simulink model "CH4_3"  (Simulink 5.0)
settings: Solver=ode23tb  SolverMode=SingleTasking  StartTime=0.0  StopTime=8/60  FixedStep=100e-6  RelTol=1e-3  AbsTol=1e-2
libraries: powerlib2 x15, powerlib_extras x6
Description:
  | 高苑科技大學 電機系
  | 電力電子實驗室
settings Model: Creator=徐瑞隆老師  LastModifiedBy=ELECTRONIC  ExtModeTrigMode=oneshot  ExtModeArmWhenConnect=off  SaveTime=off  TimeSaveName=t  SaveOutput=off  LimitDataPoints=off  BlockReductionOpt=off  BooleanDataType=off  RTWTemplateMakefile=grt_unix.tmf

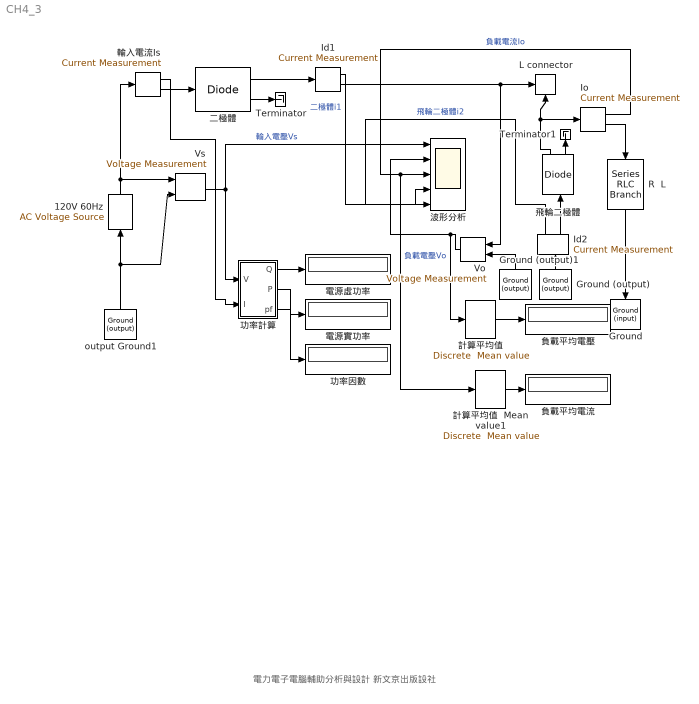
== system CH4_3 ==
  note: 電力電子電腦輔助分析與設計 新文京出版設社
  120V 60Hz : powerlib2/Electrical Sources/AC Voltage Source  Tag=PoWeRsYsTeMbLoCk  Orientation=up  A=120*1.414  P=0  F=60  stime=0  mesure=None  PSBOutputType=1
  Ground : powerlib2/Connectors/Ground (input)  Tag=PoWeRsYsTeMbLoCk  Orientation=down
  Ground (output) : powerlib2/Connectors/Ground (output)  Tag=PoWeRsYsTeMbLoCk  Orientation=up  PSBOutputType=1
  Ground (output)1 : powerlib2/Connectors/Ground (output)  Tag=PoWeRsYsTeMbLoCk  Orientation=up  PSBOutputType=1
  Id1 : powerlib2/Measurements/Current Measurement  Tag=PoWeRsYsTeMmEaSuReMeNt  PhasorSimulation=off  OutputType=Magnitude  PSBOutputType=01  PSBequivalent=0
  Id2 : powerlib2/Measurements/Current Measurement  Tag=PoWeRsYsTeMmEaSuReMeNt  Orientation=up  PhasorSimulation=off  OutputType=Magnitude  PSBOutputType=01  PSBequivalent=0
  Io : powerlib2/Measurements/Current Measurement  Tag=PoWeRsYsTeMmEaSuReMeNt  PhasorSimulation=off  OutputType=Magnitude  PSBOutputType=01  PSBequivalent=0
  L connector : powerlib2/Connectors/L connector  Tag=PoWeRsYsTeMbLoCk  Orientation=up
  R  L : powerlib2/Elements/Series RLC Branch  Tag=PoWeRsYsTeMbLoCk  Orientation=down  a=5  b=20e-03  c=inf  mesure=None  PSBOutputType=1
  Terminator : Terminator
  Terminator1 : Terminator
      settings: Orientation=up
  Vo : powerlib2/Measurements/Voltage Measurement  Tag=PoWeRsYsTeMmEaSuReMeNt  Orientation=left  PhasorSimulation=off  OutputType=Magnitude  PSBOutputType=0  PSBequivalent=0
  Vs : powerlib2/Measurements/Voltage Measurement  Tag=PoWeRsYsTeMmEaSuReMeNt  PhasorSimulation=off  OutputType=Magnitude  PSBOutputType=0  PSBequivalent=0
  output Ground1 : powerlib2/Connectors/Ground (output)  Tag=PoWeRsYsTeMbLoCk  Orientation=up  PSBOutputType=1
  二極體 : powerlib2/Power Electronics/Diode  Tag=PoWeRsYsTeMbLoCk  Ron=0.001  Lon=1e-6  Vf=0.8  IC=0  Rs=20  Cs=4e-6  PSBOutputType=10
  功率因數 : Display
  功率計算 : Subsystem
  波形分析 : Scope  NumInputPorts=5
      settings: TimeRange=0.06  YMin=-200~-200~0~-200~-5  YMax=200~200~200~200~5  DataFormat=Array
  計算平均值 : powerlib_extras/Discrete Measurements/Discrete  Mean value  AncestorBlock=|  Freq=60  Vinit=0  Ts=50e-6
      | powerlib_extras/Discrete
      | Measurements/Discrete 
      | Mean value
  計算平均值  Mean value1 : powerlib_extras/Discrete Measurements/Discrete  Mean value  AncestorBlock=|  Freq=60  Vinit=0  Ts=50e-6
      | powerlib_extras/Discrete
      | Measurements/Discrete 
      | Mean value
  負載平均電流 : Display
  負載平均電壓 : Display
  飛輪二極體 : powerlib2/Power Electronics/Diode  Tag=PoWeRsYsTeMbLoCk  Orientation=up  Ron=0.01  Lon=0  Vf=0.8  IC=0  Rs=10  Cs=0.01e-6  PSBOutputType=10
  電源虛功率 : Display
  "電源實功率 " : Display
  輸入電流Is : powerlib2/Measurements/Current Measurement  Tag=PoWeRsYsTeMmEaSuReMeNt  PhasorSimulation=off  OutputType=Magnitude  PSBOutputType=01  PSBequivalent=0
  wires:
  R  L/1 -> Ground/1
  二極體/1 -> Id1/1
  output Ground1/1 -> 120V 60Hz/1, Vs/2
  Vo/1 -> 波形分析/2, 計算平均值/1  "負載電壓Vo"
  計算平均值/1 -> 負載平均電壓/1
  計算平均值  Mean value1/1 -> 負載平均電流/1
  輸入電流Is/2 -> 二極體/1
  120V 60Hz/1 -> 輸入電流Is/1, Vs/1
  Vs/1 -> 波形分析/1, 功率計算/1(V)  "輸入電壓Vs"
  輸入電流Is/1 -> 功率計算/2(I)
  功率計算/1(Q) -> 電源虛功率/1
  功率計算/2(P) -> "電源實功率 "/1
  功率計算/3(pf) -> 功率因數/1
  Id1/2 -> L connector/Enable, Vo/1
  飛輪二極體/1 -> L connector/1, Io/1
  Ground (output)1/1 -> Vo/2
  Ground (output)/1 -> Id2/1
  Id2/2 -> 飛輪二極體/1
  Io/2 -> R  L/1
  Io/1 -> 波形分析/3, 計算平均值  Mean value1/1  "負載電流Io"
  Id2/1 -> 波形分析/4  "飛輪二極體i2"
  二極體/2 -> Terminator/1
  飛輪二極體/2 -> Terminator1/1
  Id1/1 -> 波形分析/5  "二極體i1"

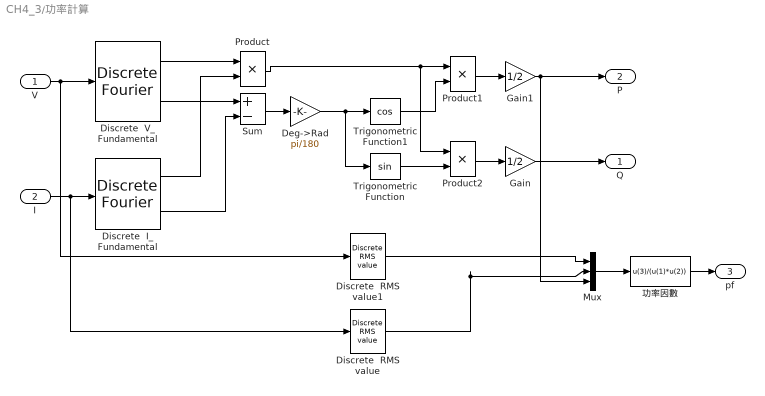
== system CH4_3/功率計算 ==
  V : Inport
  I : Inport  Port=2
  Deg->Rad : Gain  Gain=pi/180  SaturateOnIntegerOverflow=on
  Discrete  I_Fundamental : powerlib_extras/Discrete Measurements/Discrete  Fourier  Freq=60  n=1  Par_Init=[0 0]  Ts=50e-6
  Discrete  RMS value : powerlib_extras/Discrete Measurements/Discrete  RMS value  Freq=60  Mag_Init=0  Ts=50e-6
  Discrete  RMS value1 : powerlib_extras/Discrete Measurements/Discrete  RMS value  Freq=60  Mag_Init=0  Ts=50e-6
  Discrete  V_Fundamental : powerlib_extras/Discrete Measurements/Discrete  Fourier  Freq=60  n=1  Par_Init=[0 0]  Ts=50e-6
  Gain : Gain  Gain=1/2  SaturateOnIntegerOverflow=on
  Gain1 : Gain  Gain=1/2  SaturateOnIntegerOverflow=on
  Mux : Mux  Inputs=3
  Product : Product  SaturateOnIntegerOverflow=on  InputSameDT=on
  Product1 : Product  SaturateOnIntegerOverflow=on  InputSameDT=on
  Product2 : Product  SaturateOnIntegerOverflow=on  InputSameDT=on
  Sum : Sum  Inputs=+-  SaturateOnIntegerOverflow=on  InputSameDT=on
  Trigonometric Function : Trigonometry
  Trigonometric Function1 : Trigonometry  Operator=cos
  功率因數 : Fcn  Expr=u(3)/(u(1)*u(2))
  Q : Outport
  P : Outport  Port=2
  pf : Outport  Port=3
  wires:
  Gain/1 -> Q/1
  Discrete  I_Fundamental/1 -> Product/2
  Discrete  V_Fundamental/1 -> Product/1
  Trigonometric Function1/1 -> Product1/2
  Product/1 -> Product2/1, Product1/1
  Trigonometric Function/1 -> Product2/2
  Deg->Rad/1 -> Trigonometric Function/1, Trigonometric Function1/1
  Sum/1 -> Deg->Rad/1
  Discrete  I_Fundamental/2 -> Sum/2
  Discrete  V_Fundamental/2 -> Sum/1
  I/1 -> Discrete  I_Fundamental/1, Discrete  RMS value/1
  V/1 -> Discrete  V_Fundamental/1, Discrete  RMS value1/1
  Product1/1 -> Gain1/1
  Product2/1 -> Gain/1
  Gain1/1 -> P/1, Mux/3
  Mux/1 -> 功率因數/1
  功率因數/1 -> pf/1
  Discrete  RMS value1/1 -> Mux/1
  Discrete  RMS value/1 -> Mux/2
